simulink model "Utkarsh_2005574_W2_P1"  (R2020b)
settings: Solver=VariableStepAuto  StartTime=0.0  StopTime=70  RelTol=1e-3
settings Model: Creator=home  LastModifiedBy=home

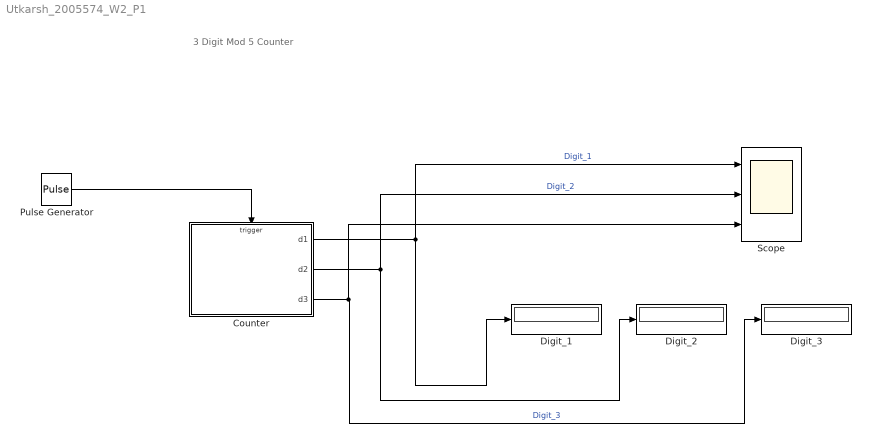
== system Utkarsh_2005574_W2_P1 ==
  note: 3 Digit Mod 5 Counter
  Counter : Stateflow chart  TreatAsAtomicUnit=on
  Digit_1 : Display
  Digit_2 : Display
  Digit_3 : Display
  Pulse Generator : DiscretePulseGenerator  PulseType=Time based  Period=1  PulseWidth=50
  Scope : Scope  NumInputPorts=3
  wires:
  Pulse Generator/1 -> Counter/Trigger
  Counter/1(d1) -> Scope/1, Digit_1/1  "Digit_1"
  Counter/2(d2) -> Digit_2/1, Scope/2  "Digit_2"
  Counter/3(d3) -> Scope/3, Digit_3/1  "Digit_3"

== stateflow chart Utkarsh_2005574_W2_P1/Counter ==
  settings: executeAtInitialization=1
  state digit1 [parallel]
    settings: executionOrder=1
    state one
      en: d1 = 1;
    state two
      en: d1 = 2;
    state three
      en: d1 = 3;
    state zero
      en: d1 = 0;
    state four
      en: d1 = 4;
    digit1.three -> digit1.four : inputClick
    digit1.zero -> digit1.one : inputClick
    digit1.two -> digit1.three : inputClick
    digit1.one -> digit1.two : inputClick
    (default) -> digit1.zero
    digit1.four -> digit1.zero : inputClick /{digit2.inc2;}
  state digit2 [parallel]
    settings: executionOrder=2
    state one
      en: d2 = 1;
    state two
      en: d2 = 2;
    state three
      en: d2 = 3;
    state zero
      en: d2 = 0;
    state four
      en: d2 = 4;
    digit2.three -> digit2.four : inc2
    digit2.zero -> digit2.one : inc2
    digit2.one -> digit2.two : inc2
    digit2.two -> digit2.three : inc2
    (default) -> digit2.zero
    digit2.four -> digit2.zero : inc2 /{digit3.inc3;}
  state digit3 [parallel]
    settings: executionOrder=3
    state one
      en: d3 = 1;
    state two
      en: d3 = 2;
    state three
      en: d3 = 3;
    state zero
      en: d3 = 0;
    state four
      en: d3 = 4;
    digit3.three -> digit3.four : inc3
    digit3.one -> digit3.two : inc3
    digit3.two -> digit3.three : inc3
    digit3.zero -> digit3.one : inc3
    digit3.four -> digit3.zero : inc3
    (default) -> digit3.zero
  data: d1 output size=1; d2 output size=1; d3 output size=1
  events: inc2 local EITHER_EDGE_EVENT; inc3 local EITHER_EDGE_EVENT; inputClick input EITHER_EDGE_EVENT
